simulink model "n"  (Simulink 8.1)
settings: Solver=ode45  StartTime=0.0  StopTime=10.0  RelTol=1e-3
settings Model: Creator=Leo  LastModifiedBy=Leo
settings DataIOCC: SignalLoggingSaveFormat=Dataset
settings OptimizationCC: ExpressionDepthLimit=128
settings DebuggingCC: FcnCallInpInsideContextMsg=EnableAllAsError
settings GRTTargetCC: CombineOutputUpdateFcns=on  GRTInterface=off

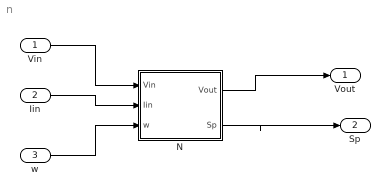
== system n ==
  Vin : Inport
  Iin : Inport  Port=2
  w : Inport  Port=3
  N : Subsystem
  Vout : Outport
  Sp : Outport  Port=2
  wires:
  Vin/1 -> N/1(Vin)
  Iin/1 -> N/2(Iin)
  w/1 -> N/3(w)
  N/1(Vout) -> Vout/1
  N/2(Sp) -> Sp/1

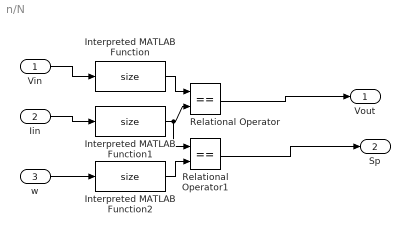
== system n/N ==
  Vin : Inport
  Iin : Inport  Port=2
  w : Inport  Port=3
  Interpreted MATLAB Function : MATLABFcn  MATLABFcn=size
  Interpreted MATLAB Function1 : MATLABFcn  MATLABFcn=size
  Interpreted MATLAB Function2 : MATLABFcn  MATLABFcn=size
  Relational Operator : RelationalOperator  Operator===  OutDataTypeStr=boolean
  Relational Operator1 : RelationalOperator  Operator===  OutDataTypeStr=boolean
  Vout : Outport
  Sp : Outport  Port=2
  wires:
  Interpreted MATLAB Function1/1 -> Relational Operator1/1, Relational Operator/2
  Iin/1 -> Interpreted MATLAB Function1/1
  Relational Operator1/1 -> Sp/1
  w/1 -> Interpreted MATLAB Function2/1
  Vin/1 -> Interpreted MATLAB Function/1
  Interpreted MATLAB Function/1 -> Relational Operator/1
  Interpreted MATLAB Function2/1 -> Relational Operator1/2
  Relational Operator/1 -> Vout/1
